simulink model "ModelRiki"  (R2020a)
settings: Solver=ode45  StartTime=0.0  StopTime=inf  MaxStep=Ts  RelTol=1e-3  EnableMultiTasking=on
model workspace (MAT data in the model file):
  CG = Simulink.Parameter
  CG.Value = [0 0 0]
  CG.DataType = 'auto'
  CG.Dimensions = [1 3]
  GPSLL = Simulink.Parameter
  GPSLL.Value = [47.255 11.345]
  GPSLL.DataType = 'auto'
  GPSLL.Dimensions = [1 2]
  Inertia = Simulink.Parameter
  Inertia.Value = [0.035  0  0; 0  0.035  0; 0  0  0.011]
  Inertia.DataType = 'auto'
  Inertia.Dimensions = [3 3]
  Mass = Simulink.Parameter
  Mass.Value = 1.6
  Mass.DataType = 'auto'
  Mass.Dimensions = [1 1]
  Ts = Simulink.Parameter
  Ts.Value = 0.0025
  Ts.DataType = 'auto'
  Ts.Dimensions = [1 1]
values from neighbouring files (symbols this model uses):
  AltKp = 0.03    [params.mat]
  AltRateBias = 0.65    [params.mat]
  AltRateKi = 0.01    [params.mat]
  AltRateKp = 0.05    [params.mat]
  AltRateMax = 6    [params.mat]
  FilterK = [0.01 0.01 0.01 0.01 0.01 0.01 0.01 0.01 0.01 0.01 0.01 0.01 ... (100 elements, 1x100)]    [params.mat]
  PosKp = 0.1    [params.mat]
  RollPitchKp = 10    [params.mat]
  RollPitchMax = 30    [params.mat]
  RollPitchRateKd = 5e-05    [params.mat]
  RollPitchRateKi = 0.002    [params.mat]
  RollPitchRateKp = 0.0007    [params.mat]
  RollPitchRateMax = 200    [params.mat]
  VelKi = 0.02    [params.mat]
  VelKp = 0.15    [params.mat]
  VelMax = 6    [params.mat]
  Waypts = [10 20 50 50 50 50 200 20 20 0 0 50 ... (27 elements, 9x3)]    [params.mat]
  YawKp = 3    [params.mat]
  YawRateKi = 0.000213867089849    [params.mat]
  YawRateKp = 0.00321759853461    [params.mat]
  YawRateMax = 180    [params.mat]
undefined symbols (not defined in the file or in its folder): AltRateKd, DiscIntNeverNeededParam, Earth, Receive, Send, sigbuilder_block, WGS84
libraries: simulink x50, sharedutil x8, simulink_extras x7, aerolibfltsims x5, aerolibanimutils x2, aerolibtransform2 x2, aerolibconvert2 x2, shared6dof x1, aerolibatmos2 x1
(part 1 of 4)
settings Model: Creator=User  LastModifiedBy=Ivan
settings SolverCC: InitialStep=Ts
settings DataIOCC: LimitDataPoints=on  SaveFormat=Array  ReturnWorkspaceOutputs=off
settings OptimizationCC: ZeroExternalMemoryAtStartup=off  ZeroInternalMemoryAtStartup=off  LifeSpan=Inf  EfficientTunableParamExpr=on
settings DebuggingCC: UnderspecifiedInitializationDetection=Classic  MergeDetectMultiDrivingBlocksExec=none  SolverPrmCheckMsg=warning  ParameterPrecisionLossMsg=none  AllowSymbolicDim=off  ModelReferenceExtraNoncontSigs=none  StateNameClashWarn=warning  SFUnexpectedBacktrackingDiag=warning  SFNoUnconditionalDefaultTransitionDiag=warning  SFExecutionAtInitializationDiag=none  ArithmeticOperatorsInVariantConditions=warning
settings HardwareCC: ProdBitPerPointer=32  ProdBitPerSizeT=32  ProdBitPerPtrDiffT=32  ProdIntDivRoundTo=Undefined  ProdWordSize=32  ProdHWDeviceType=Texas Instruments->TMS470
settings ModelReferenceCC: PropagateSignalLabelsOutOfModel=off
settings SFSimCC: SimUseLocalCustomCode=off  MATLABDynamicMemAlloc=off  CustomCodeUndefinedFunction=UseInterfaceOnly
settings RTWCC: SystemTargetFile=ert.tlc  TemplateMakefile=ert_default_tmf  GenerateReport=on  RTWUseLocalCustomCode=off  IncludeHyperlinkInReport=on  LaunchReport=on  TargetLang=C++  GenerateTraceInfo=on  GenerateTraceReport=on  GenerateTraceReportSl=on  GenerateTraceReportSf=on  GenerateTraceReportEml=on
settings CodeAppCC: StateflowObjectComments=on
settings ERTTargetCC: MultiwordLength=2048  GenerateSampleERTMain=on  MultiInstanceERTCode=on  CodeInterfacePackaging=C++ class  SupportNonFinite=off  RootIOFormat=Structure reference  ERTCustomFileTemplate=example_file_process.tlc  ConvertIfToSwitch=off  SuppressUnreachableDefaultCases=off
settings ConfigComp: CovMetricSettings=dw  CovHtmlReporting=on  CovSaveCumulativeToWorkspaceVar=on  CovSaveSingleToWorkspaceVar=on  CovExternalEMLEnable=off

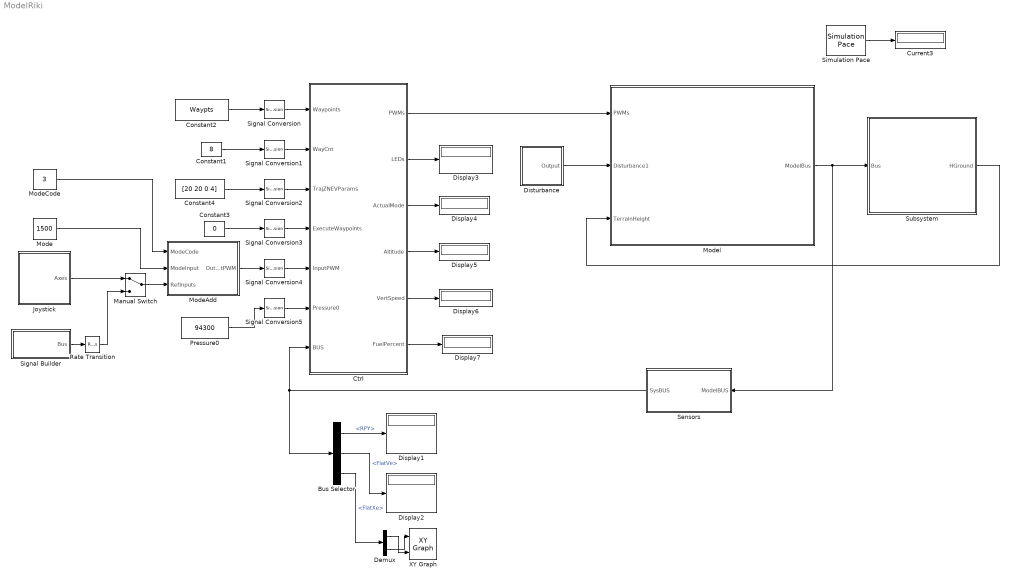
== system ModelRiki ==
  Bus Selector : BusSelector  OutputSignals=RPY,FlatVe,FlatXe
  Constant1 : Constant  Value=8  OutDataTypeStr=int32  SampleTime=Ts
  Constant2 : Constant  Value=Waypts  OutDataTypeStr=single  SampleTime=Ts
  Constant3 : Constant  Value=0  OutDataTypeStr=uint32  SampleTime=Ts
  Constant4 : Constant  Value=[20 20 0 4]  OutDataTypeStr=single  SampleTime=Ts
  Ctrl : Subsystem  TreatAsAtomicUnit=on
  Current3 : Display
  Demux : Demux  Outputs=2
  Display{1..7} (7 alike) : Display
  Disturbance : Subsystem
  Joystick : Subsystem
  Manual Switch : ManualSwitch
  Mode : Constant  Value=1500  OutDataTypeStr=uint32  SampleTime=Ts
  ModeAdd : Subsystem
  ModeCode : Constant  Value=3  OutDataTypeStr=uint8  SampleTime=Ts
  Model : Subsystem
      mask Display:
      | image('riki.jpg')
      | color('black')
      | port_label('input',1,'U')
      | port_label('input',2,'Disturbance')
      | port_label('input',3,'Terrain Height')
      | port_label('output',1,'ModelBUS')
  Pressure0 : Constant  Value=94300  OutDataTypeStr=single  SampleTime=Ts
  Rate Transition : RateTransition  OutPortSampleTime=Ts
  Sensors : Subsystem
  Signal Conversion{,1..5} (6 alike) : SignalConversion  OverrideOpt=on
  Signal Builder : Subsystem  Tag=STV Subsys  LoadFcn=sigbuilder_block('load');  StartFcn=sigbuilder_block('start');  StopFcn=sigbuilder_block('stop');  ClipboardFcn=sigbuilder_block('clipboard');  mask(Sigbuilder block){tuvar=[0:10]}
      mask help: Simulink:masks:SigbuilderBlock_MD
      mask init:
      | if ~strcmp(get_param(bdroot(gcbh),'SimulationStatus'),'stopped') tuvar = sigbuilder_block('maskInit'); end
      settings: CopyFcn=sigbuilder_block('copy');  DeleteFcn=sigbuilder_block('delete');  ModelCloseFcn=sigbuilder_block('modelClose');  PreSaveFcn=sigbuilder_block('preSave');  PauseFcn=sigbuilder_block('pause');  ContinueFcn=sigbuilder_block('continue');  NameChangeFcn=sigbuilder_block('namechange');  OpenFcn=sigbuilder_block('open',[369 90.5 830 726.5 ]);  CloseFcn=sigbuilder_block('close');
      mask Display: plot(0, 0, 100, 100,[2, 2, 32, 32, 2], [68, 8, 8, 68, 68],[32, 2], [38, 38], [32, 19, 2],[53, 60, 44], [32, 17, 17, 2],[16, 16, 31, 31]);txt = getActiveGroup(gcbh);text(2, 100, txt,'verticalAlignment', 'top');
  Simulation Pace : aerolibanimutils/Simulation Pace  SimulationPace=1  SleepMode=MATLAB Thread  OutputPaceError=on  SampleTime=Ts
      settings: AttributesFormatString=%<SimulationPace> sec/sec
  Subsystem : Subsystem
  XY Graph : simulink/Sinks/XY Graph  xmin=-100  xmax=100  ymin=-100  ymax=100  st=0.1
  wires:
  Disturbance/1(Output) -> Model/2(Disturbance1)
  Model/1(ModelBus) -> Sensors/1(ModelBUS), Subsystem/1(Bus)
  Sensors/1(SysBUS) -> Ctrl/7(BUS), Bus Selector/1
  Ctrl/1(PWMs) -> Model/1(PWMs)
  Bus Selector/1 -> Display1/1  "<RPY>"
  Ctrl/2(LEDs) -> Display3/1
  Ctrl/3(ActualMode) -> Display4/1
  Ctrl/4(Altitude) -> Display5/1
  Ctrl/5(VertSpeed) -> Display6/1
  ModeCode/1 -> ModeAdd/1(ModeCode)
  ModeAdd/1(OutputPWM) -> Signal Conversion4/1
  Subsystem/1(HGround) -> Model/3(TerrainHeight)
  Simulation Pace/1 -> Current3/1
  Bus Selector/2 -> Display2/1  "<FlatVe>"
  Mode/1 -> ModeAdd/2(ModeInput)
  Joystick/1(Axes) -> Manual Switch/1
  Manual Switch/1 -> ModeAdd/3(RefInputs)
  Constant2/1 -> Signal Conversion/1
  Constant1/1 -> Signal Conversion1/1
  Constant3/1 -> Signal Conversion3/1
  Ctrl/6(FuelPercent) -> Display7/1
  Signal Builder/1(Bus) -> Rate Transition/1
  Rate Transition/1 -> Manual Switch/2
  Demux/1 -> XY Graph/2
  Demux/2 -> XY Graph/1
  Bus Selector/3 -> Demux/1  "<FlatXe>"
  Constant4/1 -> Signal Conversion2/1
  Signal Conversion/1 -> Ctrl/1(Waypoints)
  Signal Conversion1/1 -> Ctrl/2(WayCnt)
  Signal Conversion2/1 -> Ctrl/3(TrajZNEVParams)
  Signal Conversion3/1 -> Ctrl/4(ExecuteWaypoints)
  Signal Conversion4/1 -> Ctrl/5(InputPWM)
  Pressure0/1 -> Signal Conversion5/1
  Signal Conversion5/1 -> Ctrl/6(Pressure0)

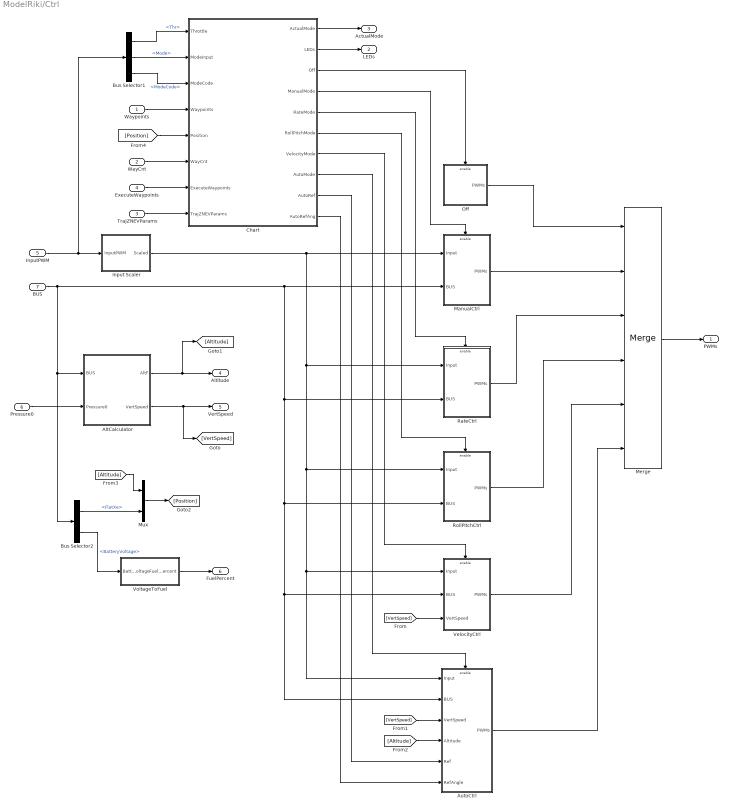
== system ModelRiki/Ctrl ==
  Waypoints : Inport
  WayCnt : Inport  Port=2
  TrajZNEVParams : Inport  Port=3
  ExecuteWaypoints : Inport  Port=4
  InputPWM : Inport  Port=5
  Pressure0 : Inport  Port=6
  BUS : Inport  Port=7
  AltCalculator : Subsystem
  AutoCtrl : Subsystem
  Bus Selector1 : BusSelector  OutputSignals=Thr,Mode,ModeCode
  Bus Selector2 : BusSelector  OutputSignals=FlatXe,BatteryVoltage
  Chart : Stateflow chart  TreatAsAtomicUnit=on
  Input Scaler : Subsystem
  ManualCtrl : Subsystem
  Merge : Merge  Inputs=6
  Mux : Mux  Inputs=2
  Off : Subsystem
  RateCtrl : Subsystem
  RollPitchCtrl : Subsystem
  VelocityCtrl : Subsystem
  VoltageToFuel : Subsystem
  PWMs : Outport
  LEDs : Outport  Port=2
  ActualMode : Outport  Port=3
  Altitude : Outport  Port=4
  VertSpeed : Outport  Port=5
  FuelPercent : Outport  Port=6
  wires:
  BUS/1 -> Bus Selector2/1, AltCalculator/1(BUS), ManualCtrl/2(BUS), RateCtrl/2(BUS), RollPitchCtrl/2(BUS), VelocityCtrl/2(BUS), AutoCtrl/2(BUS)
  InputPWM/1 -> Input Scaler/1(InputPWM), Bus Selector1/1
  Off/1(PWMs) -> Merge/1
  ManualCtrl/1(PWMs) -> Merge/2
  Merge/1 -> PWMs/1
  Chart/3(" Off") -> Off/Enable
  Chart/5(" RateMode") -> RateCtrl/Enable
  Bus Selector1/1 -> Chart/1(Throttle)  "<Thr>"
  Input Scaler/1(Scaled) -> ManualCtrl/1(Input), RateCtrl/1(Input), RollPitchCtrl/1(Input), AutoCtrl/1(Input), VelocityCtrl/1(Input)
  Chart/1(ActualMode) -> ActualMode/1
  Chart/6(" RollPitchMode") -> RollPitchCtrl/Enable
  Chart/2(LEDs) -> LEDs/1
  RollPitchCtrl/1(PWMs) -> Merge/4
  Chart/4(" ManualMode") -> ManualCtrl/Enable
  RateCtrl/1(PWMs) -> Merge/3
  AltCalculator/1(AltF) -> [Altitude], Altitude/1
  AltCalculator/2(VertSpeed) -> [VertSpeed], VertSpeed/1
  Bus Selector1/3 -> Chart/3(ModeCode)  "<ModeCode>"
  VelocityCtrl/1(PWMs) -> Merge/5
  Chart/7(" VelocityMode") -> VelocityCtrl/Enable
  AutoCtrl/1(PWMs) -> Merge/6
  Bus Selector1/2 -> Chart/2(ModeInput)  "<Mode>"
  [VertSpeed] -> VelocityCtrl/3(VertSpeed)
  [VertSpeed] -> AutoCtrl/3(VertSpeed)
  [Altitude] -> AutoCtrl/4(Altitude)
  Waypoints/1 -> Chart/4(Waypoints)
  Bus Selector2/1 -> Mux/2  "<FlatXe>"
  [Altitude] -> Mux/1
  Mux/1 -> [Position]
  [Position] -> Chart/5(Position)
  WayCnt/1 -> Chart/6(WayCnt)
  ExecuteWaypoints/1 -> Chart/7(ExecuteWaypoints)
  Bus Selector2/2 -> VoltageToFuel/1(BattVoltage)  "<BatteryVoltage>"
  VoltageToFuel/1(FuelPercent) -> FuelPercent/1
  Pressure0/1 -> AltCalculator/2(Pressure0)
  Chart/10(AutoRefAng) -> AutoCtrl/6(RefAngle)
  TrajZNEVParams/1 -> Chart/8(TrajZNEVParams)
  Chart/8(" AutoMode") -> AutoCtrl/Enable
  Chart/9(AutoRef) -> AutoCtrl/5(Ref)

== system ModelRiki/Disturbance ==
  Mode3 : Constant  Value=[0 0 0]  OutDataTypeStr=Inherit: Inherit via back propagation  SampleTime=Ts
  Mux : Mux  Inputs=2
  Step : Step  Time=10  Before=[0 0 0]  After=[0 0 0]  SampleTime=0
  Output : Outport
  wires:
  Step/1 -> Mux/1  "F[N]"
  Mux/1 -> Output/1
  Mode3/1 -> Mux/2  "Torque"

== system ModelRiki/Joystick ==
  Bus Creator : BusCreator  Inputs=4
  Joy Scaler : Subsystem
  Joystick : Subsystem
  Terminator{,1..3} (4 alike) : Terminator
  Axes : Outport
  wires:
  Joystick/1(Roll) -> Bus Creator/1  "Roll"
  Joystick/2(Pitch) -> Bus Creator/2  "Pitch"
  Joystick/3(Yaw) -> Bus Creator/3  "Yaw"
  Joystick/4(Throttle) -> Bus Creator/4  "Throttle"
  Bus Creator/1 -> Joy Scaler/1(Joystick)
  Joystick/7(B3) -> Terminator3/1
  Joystick/6(B2) -> Terminator1/1
  Joystick/5(B1) -> Terminator/1
  Joystick/8(B4) -> Terminator2/1
  Joy Scaler/1(Scaled) -> Axes/1

== system ModelRiki/ModeAdd ==
  ModeCode : Inport
  ModeInput : Inport  Port=2
  RefInputs : Inport  Port=3
  Bus Creator : BusCreator  Inputs=6
  Bus Selector2 : BusSelector  OutputSignals=Thr,Aileron,Elevator,Rudder
  Data Type Conversion{,1..3} (4 alike) : DataTypeConversion  OutDataTypeStr=single
  OutputPWM : Outport
  wires:
  Bus Selector2/1 -> Data Type Conversion/1  "<Thr>"
  Bus Selector2/2 -> Data Type Conversion1/1  "<Aileron>"
  RefInputs/1 -> Bus Selector2/1
  Bus Selector2/3 -> Data Type Conversion2/1  "<Elevator>"
  Bus Selector2/4 -> Data Type Conversion3/1  "<Rudder>"
  ModeCode/1 -> Bus Creator/1  "ModeCode"
  Bus Creator/1 -> OutputPWM/1
  ModeInput/1 -> Bus Creator/2  "Mode"
  Data Type Conversion/1 -> Bus Creator/3  "Thr"
  Data Type Conversion1/1 -> Bus Creator/4  "Aileron"
  Data Type Conversion2/1 -> Bus Creator/5  "Elevator"
  Data Type Conversion3/1 -> Bus Creator/6  "Rudder"

== system ModelRiki/Model ==
  note: DCM:
      | Pbody = DCM*Pearth
  PWMs : Inport
  Disturbance1 : Inport  Port=2
  TerrainHeight : Inport  Port=3
  6DoF (Euler Angles) : shared6dof/6DOF (Euler Angles)  units=Metric (MKS)  mtype=Fixed  rep=Euler Angles  xme_0=[0 0 -600]  Vm_0=[0 0 0]  eul_0=[0 0 0]  pm_0=[0 0 0]  mass_0=Mass  mass_e=0.5  mass_f=2.0  inertia=Inertia  inertia_e=eye(3)  inertia_f=2*eye(3)  k_quat=1.0  vre_flag=on  abi_flag=off  aMode=aMode  xme_statename=''  Vm_statename=''  eul_statename=''  quat_statename=''  pm_statename=''  mass_statename=''
      settings: SourceProductBaseCode=AE,PW,MT,VE,VP
  Bus Creator : BusCreator  Inputs=10
  Bus Selector : BusSelector  OutputSignals=PWM1,PWM2,PWM3,PWM4
  Environment : Subsystem
  GPS&Pressure : Subsystem
  Ground : Ground
  Landing Gears : Subsystem
  Manual Switch1 : ManualSwitch
  Propulsion : Subsystem
  Rate Transition : RateTransition
  Sum : Sum  Inputs=||+-+
  Sum1 : Sum  Inputs=||+-+
  Terminator1 : Terminator
  Terminator2 : Terminator
  ModelBus : Outport
  wires:
  6DoF (Euler Angles)/1 -> Bus Creator/1  "Ve"
  6DoF (Euler Angles)/2 -> GPS&Pressure/1(Xe), Bus Creator/2  "Xe"
  6DoF (Euler Angles)/3 -> Bus Creator/3  "RPY"
  6DoF (Euler Angles)/4 -> Bus Creator/4  "DCM"
  Propulsion/2(Mxyz[Nm]) -> Sum1/1
  Propulsion/1(Fxyz[N]) -> Sum/1
  6DoF (Euler Angles)/7 -> Terminator2/1
  Sum/1 -> Manual Switch1/1
  Ground/1 -> Manual Switch1/2
  PWMs/1 -> Rate Transition/1
  Bus Selector/1 -> Propulsion/1(PWM1)  "<PWM1>"
  Bus Selector/2 -> Propulsion/2(PWM2)  "<PWM2>"
  Bus Selector/3 -> Propulsion/3(PWM3)  "<PWM3>"
  Bus Selector/4 -> Propulsion/4(PWM4)  "<PWM4>"
  Manual Switch1/1 -> 6DoF (Euler Angles)/1
  6DoF (Euler Angles)/5 -> Bus Creator/5  "Vb"
  6DoF (Euler Angles)/6 -> Bus Creator/6  "dRPY"
  Rate Transition/1 -> Bus Selector/1
  6DoF (Euler Angles)/8 -> Terminator1/1  "Accel"
  GPS&Pressure/1(GpsLL) -> Bus Creator/7  "GpsLL"
  GPS&Pressure/2(GPSHeight) -> Bus Creator/8  "GpsHeight"
  GPS&Pressure/3(PressurePa) -> Bus Creator/9  "PressurePa"
  Bus Creator/1 -> Landing Gears/1(Model Bus), Environment/1(Model Bus), ModelBus/1
  Propulsion/3(TotalCurrent[A]) -> Bus Creator/10  "TotalCurrent"
  Disturbance1/1 -> Environment/2(Disturbance)
  Sum1/1 -> 6DoF (Euler Angles)/2
  Landing Gears/1(M[Nm]) -> Sum1/3
  Landing Gears/2(F[N]) -> Sum/3
  Environment/1(M[Nm]) -> Sum1/2
  Environment/2(F[N]) -> Sum/2
  TerrainHeight/1 -> Landing Gears/2(TerrainHeight)

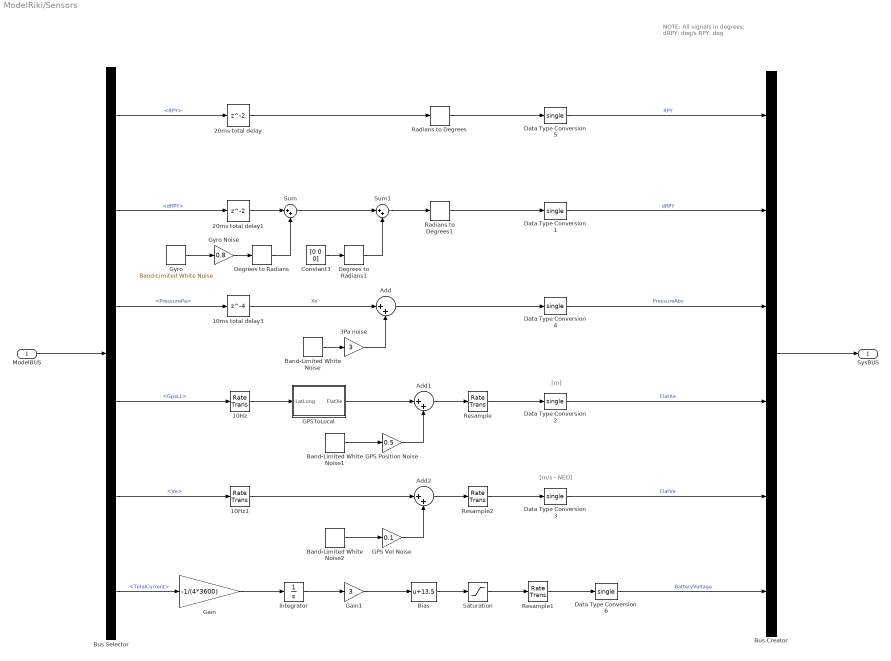
== system ModelRiki/Sensors ==
  note: [m/s - NED]
  note: [m]
  note: NOTE: All signals in degrees:
      | dRPY: deg/s
      | RPY: deg
  ModelBUS : Inport
  10Hz : RateTransition  OutPortSampleTime=1/10
  10Hz1 : RateTransition  OutPortSampleTime=1/10
  10ms total delay3 : Delay  DelayLength=4  SampleTime=Ts
  20ms total delay : Delay  SampleTime=Ts
  20ms total delay1 : Delay  SampleTime=Ts
  3Pa noise : Gain  Gain=3
  Add : Sum  Inputs=|++
  Add1 : Sum  Inputs=|++
  Add2 : Sum  Inputs=|++
  Band-Limited White Noise : simulink/Sources/Band-Limited White Noise  Cov=[1]*Ts  Ts=Ts  seed=[23341]
  Band-Limited White Noise1 : simulink/Sources/Band-Limited White Noise  Cov=[1]*Ts  Ts=Ts  seed=[23341]
  Band-Limited White Noise2 : simulink/Sources/Band-Limited White Noise  Cov=[1]*Ts  Ts=Ts  seed=[23341]
  Bias : Bias  Bias=13.5
  Bus Creator : BusCreator  Inputs=6
  Bus Selector : BusSelector  OutputSignals=RPY,dRPY,PressurePa,GpsLL,Ve,TotalCurrent
  Constant3 : Constant  Value=[0 0 0]  OutDataTypeStr=single
  Data Type Conversion{1..6} (6 alike) : DataTypeConversion  OutDataTypeStr=single
  Degrees to Radians : simulink_extras/Transformations/Degrees to Radians
  Degrees to Radians1 : simulink_extras/Transformations/Degrees to Radians
  GPS Position Noise : Gain  Gain=0.5
  GPS Vel Noise : Gain  Gain=0.1
  GPSToLocal : Subsystem
  Gain : Gain  Gain=-1/(4*3600)
  Gain1 : Gain  Gain=3
  Gyro : simulink/Sources/Band-Limited White Noise  Cov=[1]*Ts  Ts=Ts  seed=[23341]
  Gyro Noise : Gain  Gain=0.8
  Integrator : Integrator  InitialCondition=1  LimitOutput=on  UpperSaturationLimit=1  LowerSaturationLimit=0
  Radians to Degrees : simulink_extras/Transformations/Radians to Degrees
  Radians to Degrees1 : simulink_extras/Transformations/Radians to Degrees
  Resample : RateTransition  OutPortSampleTime=Ts
  Resample1 : RateTransition  OutPortSampleTime=Ts
  Resample2 : RateTransition  OutPortSampleTime=Ts
  Saturation : Saturate  UpperLimit=16.8  LowerLimit=12
  Sum : Sum  Inputs=|++
  Sum1 : Sum  Inputs=|++
  SysBUS : Outport
  wires:
  ModelBUS/1 -> Bus Selector/1
  Bus Selector/1 -> 20ms total delay/1  "<RPY>"
  Bus Creator/1 -> SysBUS/1
  Bus Selector/2 -> 20ms total delay1/1  "<dRPY>"
  20ms total delay/1 -> Radians to Degrees/1
  20ms total delay1/1 -> Sum/1
  Gyro/1 -> Gyro Noise/1
  Data Type Conversion5/1 -> Bus Creator/1  "RPY"
  Data Type Conversion1/1 -> Bus Creator/2  "dRPY"
  Degrees to Radians/1 -> Sum/2
  Radians to Degrees/1 -> Data Type Conversion5/1
  Radians to Degrees1/1 -> Data Type Conversion1/1
  Sum/1 -> Sum1/1
  Sum1/1 -> Radians to Degrees1/1
  Constant3/1 -> Degrees to Radians1/1
  Degrees to Radians1/1 -> Sum1/2
  Data Type Conversion3/1 -> Bus Creator/5  "FlatVe"
  Data Type Conversion2/1 -> Bus Creator/4  "FlatXe"
  3Pa noise/1 -> Add/2
  Band-Limited White Noise/1 -> 3Pa noise/1
  Add/1 -> Data Type Conversion4/1
  10ms total delay3/1 -> Add/1  "Xe"
  Bus Selector/3 -> 10ms total delay3/1  "<PressurePa>"
  Data Type Conversion4/1 -> Bus Creator/3  "PressureAbs"
  Bus Selector/4 -> 10Hz/1  "<GpsLL>"
  Bus Selector/5 -> 10Hz1/1  "<Ve>"
  10Hz/1 -> GPSToLocal/1(LatLong)
  Resample/1 -> Data Type Conversion2/1
  Resample2/1 -> Data Type Conversion3/1
  GPS Position Noise/1 -> Add1/2
  Band-Limited White Noise1/1 -> GPS Position Noise/1
  GPSToLocal/1(FlatXe) -> Add1/1
  Add1/1 -> Resample/1
  GPS Vel Noise/1 -> Add2/2
  Band-Limited White Noise2/1 -> GPS Vel Noise/1
  10Hz1/1 -> Add2/1
  Add2/1 -> Resample2/1
  Gyro Noise/1 -> Degrees to Radians/1
  Bus Selector/6 -> Gain/1  "<TotalCurrent>"
  Gain/1 -> Integrator/1
  Integrator/1 -> Gain1/1
  Bias/1 -> Saturation/1
  Gain1/1 -> Bias/1
  Saturation/1 -> Resample1/1
  Resample1/1 -> Data Type Conversion6/1
  Data Type Conversion6/1 -> Bus Creator/6  "BatteryVoltage"

== system ModelRiki/Signal Builder ==
  Bus Creator : BusCreator  Tag=Bus Creator  Inputs=4
  FromWs : FromWorkspace  Tag=STV FromWs  VariableName=tuvar
      SigBuilderData=|
      | common.afterFinalStr = 'Extrapolate'
      | common.sampleTime = 0
      | dataSet.timeRange = [0 20]
      | dataSet.name = 'Group 1'
      | sbobj.Groups.Name = 'Group 1'
      | sbobj.Groups.Signals(1).Name = 'Thr'
      | sbobj.Groups.Signals(1).XData = [0 20]
      | sbobj.Groups.Signals(1).YData = [1430 1430]
      | sbobj.Groups.Signals(2).Name = 'Aileron'
      | sbobj.Groups.Signals(2).XData = [0 20]
      | sbobj.Groups.Signals(2).YData = [1024 1024]
      | sbobj.Groups.Signals(3).Name = 'Elevator'
      | sbobj.Groups.Signals(3).XData = [0 20]
      | sbobj.Groups.Signals(3).YData = [1000 1000]
      | sbobj.Groups.Signals(4).Name = 'Rudder'
      | sbobj.Groups.Signals(4).XData = [0 20]
      | sbobj.Groups.Signals(4).YData = [1024 1024]
      | sbobj.Groups.TimeRange = [0 20]
  Subsystem : Subsystem
  Bus : Outport
  wires:
  FromWs/1 -> Subsystem/1(In1)
  Subsystem/1(Thr) -> Bus Creator/1  "Thr"
  Subsystem/2(Aileron) -> Bus Creator/2  "Aileron"
  Subsystem/3(Elevator) -> Bus Creator/3  "Elevator"
  Subsystem/4(Rudder) -> Bus Creator/4  "Rudder"
  Bus Creator/1 -> Bus/1

== system ModelRiki/Subsystem ==
  Bus : Inport
  Angle Conversion1 : aerolibconvert2/Angle Conversion  IU=deg  OU=rad
  Angle Conversion2 : aerolibconvert2/Angle Conversion  IU=deg  OU=rad
  Bus Selector1 : BusSelector  OutputSignals=GpsLL,GpsHeight,RPY
  Data Type Conversion1 : DataTypeConversion  OutDataTypeStr=single
  Data Type Conversion2 : DataTypeConversion  OutDataTypeStr=single
  Data Type Conversion3 : DataTypeConversion  OutDataTypeStr=single
  Demux : Demux  Outputs=2
  Demux1 : Demux  Outputs=3
  Generate Run Script : aerolibfltsims/Generate Run Script  Architecture=Win64  dataFlow=Send-Receive  GeometryModelName=Kiki  AirportId=LDZA  RunwayId=16  InitialAltitude=5000  InitialHeading=0  OffsetDistance=0  OffsetAzimuth=0  InstallScenery=off  DisableShaders=off  OriginAddress=127.0.0.1  DestinationPort=5502  OriginPort=5505  LocalAddress=127.0.0.1  OutputFileName=runfg.bat  FlightGearBaseDirectory=C:\Program Files\FlightGear 3.4.0
  Pack net_fdm Packet for FlightGear : aerolibfltsims/Pack net_fdm Packet for FlightGear  FlightGearVersion=v3.4  ShowPositionAttitudeInputs=on  ShowVelocityAccelerationInputs=off  ShowControlSurfacePositionInputs=off  ShowEngineFuelInputs=off  ShowLandingGearInputs=off  ShowEnvironmentInputs=off  SampleTime=1/30  packetVersion=24
      settings: SourceProductBaseCode=AE
  Receive net_ctrl Packet from FlightGear : aerolibfltsims/Receive net_ctrl Packet from FlightGear  FlightGearVersion=v3.4  ReceiveAddress=127.0.0.1  ReceivePort=5505  ReceiveWidth=744  varLen=off  SampleTime=1/30  packetFlag=off
      settings: AttributesFormatString=Version Selected:\n%<FlightGearVersion>  SourceProductBaseCode=AE
  Send net_fdm Packet to FlightGear : aerolibfltsims/Send net_fdm Packet to FlightGear  DestinationIpAddress=127.0.0.1  DestinationPort=5502  LocalIpPort=-1  varLen=off  SampleTime=1/30
      settings: SourceProductBaseCode=AE
  Terminator{,1..6} (7 alike) : Terminator
  Unpack net_ctrl Packet from FlightGear : aerolibfltsims/Unpack net_ctrl Packet from FlightGear  FlightGearVersion=v3.4  ShowControlSurfacePositionOutputs=off  ShowEngineFuelOutputs=off  ShowLandingGearOutputs=off  ShowAvionicOutputs=off  ShowEnvironmentOutputs=on  SampleTime=1/30  packetVersion=27
      settings: AttributesFormatString=Version Selected: %<FlightGearVersion>  SourceProductBaseCode=AE
  HGround : Outport
  wires:
  Pack net_fdm Packet for FlightGear/1 -> Send net_fdm Packet to FlightGear/1
  Bus/1 -> Bus Selector1/1
  Bus Selector1/1 -> Demux/1  "<GpsLL>"
  Demux/1 -> Angle Conversion1/1
  Demux/2 -> Angle Conversion2/1
  Bus Selector1/2 -> Pack net_fdm Packet for FlightGear/3  "<GpsHeight>"
  Demux1/1 -> Data Type Conversion1/1
  Demux1/2 -> Data Type Conversion2/1
  Demux1/3 -> Data Type Conversion3/1
  Data Type Conversion1/1 -> Pack net_fdm Packet for FlightGear/4
  Data Type Conversion2/1 -> Pack net_fdm Packet for FlightGear/5
  Data Type Conversion3/1 -> Pack net_fdm Packet for FlightGear/6
  Bus Selector1/3 -> Demux1/1  "<RPY>"
  Receive net_ctrl Packet from FlightGear/1 -> Unpack net_ctrl Packet from FlightGear/1
  Unpack net_ctrl Packet from FlightGear/6 -> HGround/1
  Angle Conversion1/1 -> Pack net_fdm Packet for FlightGear/2
  Angle Conversion2/1 -> Pack net_fdm Packet for FlightGear/1
  Unpack net_ctrl Packet from FlightGear/1 -> Terminator/1
  Unpack net_ctrl Packet from FlightGear/2 -> Terminator1/1
  Unpack net_ctrl Packet from FlightGear/3 -> Terminator2/1
  Unpack net_ctrl Packet from FlightGear/4 -> Terminator3/1
  Unpack net_ctrl Packet from FlightGear/5 -> Terminator4/1
  Unpack net_ctrl Packet from FlightGear/7 -> Terminator5/1
  Unpack net_ctrl Packet from FlightGear/8 -> Terminator6/1

== system ModelRiki/Ctrl/AltCalculator ==
  BUS : Inport
  Pressure0 : Inport  Port=2
  Bus Selector1 : BusSelector  OutputSignals=PressureAbs
  Delay : Delay  DelayLength=100
  Discrete FIR Filter : DiscreteFir  Coefficients=FilterK
  Gain : Gain  Gain=1/(100*Ts)
  MATLAB Function : MATLAB Function  TreatAsAtomicUnit=on
  Sum : Sum  Inputs=|+-
  AltF : Outport
  VertSpeed : Outport  Port=2
  wires:
  BUS/1 -> Bus Selector1/1
  Bus Selector1/1 -> MATLAB Function/1(pressure)  "<PressureAbs>"
  MATLAB Function/1(alt) -> Discrete FIR Filter/1
  Sum/1 -> Gain/1
  Discrete FIR Filter/1 -> Delay/1, Sum/1, AltF/1
  Delay/1 -> Sum/2
  Gain/1 -> VertSpeed/1
  Pressure0/1 -> MATLAB Function/2(pressure0)

== system ModelRiki/Ctrl/AutoCtrl ==
  Input : Inport  OutDataTypeStr=single
  BUS : Inport  Port=2  OutDataTypeStr=single
  VertSpeed : Inport  Port=3  OutDataTypeStr=single
  Altitude : Inport  Port=4  OutDataTypeStr=single
  Ref : Inport  Port=5  OutDataTypeStr=single
  RefAngle : Inport  Port=6  OutDataTypeStr=single
  Enable : EnablePort  StatesWhenEnabling=reset
  Alt Controller : Subsystem
  Bus Selector1 : BusSelector  OutputSignals=Rudder
  Demux : Demux  Outputs=3
  Mapper : Subsystem
  Pitch Controller : Subsystem
  Position Ctrl : Subsystem
  Roll Controller : Subsystem
  Velocity Ctrl : Subsystem
  Yaw Controller : Subsystem
  PWMs : Outport
  wires:
  BUS/1 -> Yaw Controller/1(BUS), Pitch Controller/1(BUS), Position Ctrl/1(BUS), Roll Controller/1(BUS), Velocity Ctrl/1(BUS)
  Input/1 -> Bus Selector1/1
  Bus Selector1/1 -> Yaw Controller/2(YawRef)  "<Rudder>"
  Mapper/1(Out1) -> PWMs/1
  Roll Controller/1(RollPWM) -> Mapper/2(Aileron)
  Pitch Controller/1(PitchPWM) -> Mapper/3(Elevator)
  Yaw Controller/1(YawPWM) -> Mapper/4(Rudder)
  Velocity Ctrl/1(RollRef) -> Roll Controller/2(RollRef)  "RollRef"
  Velocity Ctrl/2(PitchRef) -> Pitch Controller/2(PitchRef)  "PitchRef"
  VertSpeed/1 -> Alt Controller/2(VertVel)
  Alt Controller/1(Thrust) -> Mapper/1(Thr)
  Altitude/1 -> Alt Controller/3(Altitude)
  Position Ctrl/1(VeXref) -> Velocity Ctrl/2(VeXref)
  Position Ctrl/2(VeYRef) -> Velocity Ctrl/3(VeYref)
  Demux/2 -> Position Ctrl/2(XeXRef)
  Demux/3 -> Position Ctrl/3(XeYRef)
  Ref/1 -> Demux/1
  Demux/1 -> Alt Controller/1(AltRef)
  RefAngle/1 -> Yaw Controller/3(RefAngle)

== system ModelRiki/Ctrl/Input Scaler ==
  InputPWM : Inport
  Bus Creator : BusCreator  Inputs=4
  Bus Selector2 : BusSelector  OutputSignals=Thr,Aileron,Elevator,Rudder
  Constant : Constant  Value=350  OutDataTypeStr=single
  Constant1 : Constant  Value=1024  OutDataTypeStr=single
  Constant2 : Constant  Value=1024  OutDataTypeStr=single
  Constant3 : Constant  Value=1024  OutDataTypeStr=single
  Gain : Gain  Gain=1/(1700-350)
  Gain1 : Gain  Gain=-1/(1700-1024)
  Gain2 : Gain  Gain=-1/(1700-1024)
  Gain3 : Gain  Gain=-1/(1700-1024)
  Saturation : Saturate  UpperLimit=1  LowerLimit=0
  Saturation1 : Saturate  UpperLimit=1  LowerLimit=-1
  Saturation2 : Saturate  UpperLimit=1  LowerLimit=-1
  Saturation3 : Saturate  UpperLimit=1  LowerLimit=-1
  Subtract{,1..3} (4 alike) : Sum  Inputs=+-
  Scaled : Outport
  wires:
  Bus Creator/1 -> Scaled/1
  InputPWM/1 -> Bus Selector2/1
  Bus Selector2/1 -> Subtract/1  "<Thr>"
  Constant/1 -> Subtract/2
  Subtract/1 -> Gain/1
  Gain/1 -> Saturation/1
  Saturation/1 -> Bus Creator/1  "Thr"
  Bus Selector2/2 -> Subtract1/1  "<Aileron>"
  Constant1/1 -> Subtract1/2
  Subtract1/1 -> Gain1/1
  Gain1/1 -> Saturation1/1
  Saturation1/1 -> Bus Creator/2  "Aileron"
  Bus Selector2/3 -> Subtract2/1  "<Elevator>"
  Constant2/1 -> Subtract2/2
  Subtract2/1 -> Gain2/1
  Gain2/1 -> Saturation2/1
  Saturation2/1 -> Bus Creator/3  "Elevator"
  Bus Selector2/4 -> Subtract3/1  "<Rudder>"
  Constant3/1 -> Subtract3/2
  Subtract3/1 -> Gain3/1
  Gain3/1 -> Saturation3/1
  Saturation3/1 -> Bus Creator/4  "Rudder"

== system ModelRiki/Ctrl/ManualCtrl ==
  Input : Inport  OutDataTypeStr=single
  BUS : Inport  Port=2  OutDataTypeStr=single
  Enable : EnablePort  StatesWhenEnabling=reset
  Bus Selector1 : BusSelector  OutputSignals=Thr,Aileron,Elevator,Rudder
  Gain : Gain
  Gain1 : Gain  Gain=0.2
  Gain2 : Gain  Gain=0.2
  Gain3 : Gain  Gain=0.2
  Mapper : Subsystem
  Terminator : Terminator
  PWMs : Outport
  wires:
  Bus Selector1/4 -> Gain3/1  "<Rudder>"
  Input/1 -> Bus Selector1/1
  Bus Selector1/1 -> Gain/1  "<Thr>"
  Bus Selector1/3 -> Gain2/1  "<Elevator>"
  Bus Selector1/2 -> Gain1/1  "<Aileron>"
  BUS/1 -> Terminator/1
  Gain/1 -> Mapper/1(Thr)
  Gain1/1 -> Mapper/2(Aileron)
  Gain2/1 -> Mapper/3(Elevator)
  Gain3/1 -> Mapper/4(Rudder)
  Mapper/1(Out1) -> PWMs/1

== system ModelRiki/Ctrl/Off ==
  Enable : EnablePort  StatesWhenEnabling=reset
  Bus Creator : BusCreator  Inputs=4
  Constant{1..4} (4 alike) : Constant  Value=1000  OutDataTypeStr=single  SampleTime=Ts
  PWMs : Outport  InitialOutput=[1000 1000 1000 1000]
  wires:
  Bus Creator/1 -> PWMs/1
  Constant2/1 -> Bus Creator/1  "PWM1"
  Constant1/1 -> Bus Creator/2  "PWM2"
  Constant4/1 -> Bus Creator/4  "PWM4"
  Constant3/1 -> Bus Creator/3  "PWM3"

== system ModelRiki/Ctrl/RateCtrl ==
  Input : Inport  OutDataTypeStr=single
  BUS : Inport  Port=2  OutDataTypeStr=single
  Enable : EnablePort  StatesWhenEnabling=reset
  Bus Selector1 : BusSelector  OutputSignals=Thr,Aileron,Elevator,Rudder
  Gain : Gain
  Mapper : Subsystem
  Pitch Controller : Subsystem
  Roll Controller : Subsystem
  Yaw Controller : Subsystem
  PWMs : Outport
  wires:
  Bus Selector1/4 -> Yaw Controller/2(YawRef)  "<Rudder>"
  Input/1 -> Bus Selector1/1
  Bus Selector1/1 -> Gain/1  "<Thr>"
  Bus Selector1/3 -> Pitch Controller/2(PitchRef)  "<Elevator>"
  Bus Selector1/2 -> Roll Controller/2(RollRef)  "<Aileron>"
  BUS/1 -> Roll Controller/1(BUS), Pitch Controller/1(BUS), Yaw Controller/1(BUS)
  Mapper/1(Out1) -> PWMs/1
  Gain/1 -> Mapper/1(Thr)
  Roll Controller/1(RollPWM) -> Mapper/2(Aileron)
  Pitch Controller/1(PitchPWM) -> Mapper/3(Elevator)
  Yaw Controller/1(YawPWM) -> Mapper/4(Rudder)

== system ModelRiki/Ctrl/RollPitchCtrl ==
  Input : Inport  OutDataTypeStr=single
  BUS : Inport  Port=2  OutDataTypeStr=single
  Enable : EnablePort  StatesWhenEnabling=reset
  Bus Selector1 : BusSelector  OutputSignals=Thr,Aileron,Elevator,Rudder
  Gain : Gain
  Mapper : Subsystem
  Pitch Controller : Subsystem
  Roll Controller : Subsystem
  Yaw Controller : Subsystem
  PWMs : Outport
  wires:
  Bus Selector1/4 -> Yaw Controller/2(YawRef)  "<Rudder>"
  Input/1 -> Bus Selector1/1
  Bus Selector1/1 -> Gain/1  "<Thr>"
  Bus Selector1/3 -> Pitch Controller/2(PitchRef)  "<Elevator>"
  Bus Selector1/2 -> Roll Controller/2(RollRef)  "<Aileron>"
  BUS/1 -> Roll Controller/1(BUS), Yaw Controller/1(BUS), Pitch Controller/1(BUS)
  Mapper/1(Out1) -> PWMs/1
  Gain/1 -> Mapper/1(Thr)
  Roll Controller/1(RollPWM) -> Mapper/2(Aileron)
  Pitch Controller/1(PitchPWM) -> Mapper/3(Elevator)
  Yaw Controller/1(YawPWM) -> Mapper/4(Rudder)

== system ModelRiki/Ctrl/VelocityCtrl ==
  Input : Inport  OutDataTypeStr=single
  BUS : Inport  Port=2  OutDataTypeStr=single
  VertSpeed : Inport  Port=3  OutDataTypeStr=single
  Enable : EnablePort  StatesWhenEnabling=reset
  Alt Controller : Subsystem
  Bus Selector1 : BusSelector  OutputSignals=Thr,Elevator,Aileron,Rudder
  Gain2 : Gain  Gain=-1
  Mapper : Subsystem
  Pitch Controller : Subsystem
  Roll Controller : Subsystem
  Velocity Ctrl1 : Subsystem
  Yaw Controller : Subsystem
  PWMs : Outport
  wires:
  BUS/1 -> Velocity Ctrl1/1(BUS), Yaw Controller/1(BUS), Pitch Controller/1(BUS), Roll Controller/1(BUS)
  Input/1 -> Bus Selector1/1
  Bus Selector1/4 -> Yaw Controller/2(YawRef)  "<Rudder>"
  Roll Controller/1(RollPWM) -> Mapper/2(Aileron)
  Pitch Controller/1(PitchPWM) -> Mapper/3(Elevator)
  Yaw Controller/1(YawPWM) -> Mapper/4(Rudder)
  Bus Selector1/3 -> Velocity Ctrl1/3(VeYref)  "<Aileron>"
  Bus Selector1/2 -> Gain2/1  "<Elevator>"
  Velocity Ctrl1/1(RollRef) -> Roll Controller/2(RollRef)  "RollRef"
  Velocity Ctrl1/2(PitchRef) -> Pitch Controller/2(PitchRef)  "PitchRef"
  Gain2/1 -> Velocity Ctrl1/2(VeXref)
  Bus Selector1/1 -> Alt Controller/1(VertVellRef)  "<Thr>"
  VertSpeed/1 -> Alt Controller/2(VertVel)
  Alt Controller/1(Thrust) -> Mapper/1(Thr)
  Mapper/1(Out1) -> PWMs/1

== system ModelRiki/Ctrl/VoltageToFuel ==
  BattVoltage : Inport
  Polynomial : Polyval  Coefs=[-20.235749769635976 666.2775704118918 -5384.291364540743]
  Saturation : Saturate  UpperLimit=16.5  LowerLimit=14
  Saturation1 : Saturate  UpperLimit=100  LowerLimit=0
  FuelPercent : Outport
  wires:
  BattVoltage/1 -> Saturation/1
  Polynomial/1 -> Saturation1/1
  Saturation1/1 -> FuelPercent/1
  Saturation/1 -> Polynomial/1

== system ModelRiki/Joystick/Joy Scaler ==
  Joystick : Inport
  Bus Creator : BusCreator  Inputs=4
  Bus Selector2 : BusSelector  OutputSignals=Throttle,Roll,Pitch,Yaw
  Constant : Constant  Value=350  OutDataTypeStr=single
  Constant1 : Constant  Value=1024  OutDataTypeStr=single
  Constant2 : Constant  Value=1024  OutDataTypeStr=single
  Constant3 : Constant  Value=1024  OutDataTypeStr=single
  Gain : Gain  Gain=(1700-350)
  Gain1 : Gain  Gain=-(1024-350)
  Gain2 : Gain  Gain=-(1024-350)
  Gain3 : Gain  Gain=-(1024-350)
  Saturation{,1..3} (4 alike) : Saturate  UpperLimit=1700  LowerLimit=350  OutDataTypeStr=Inherit: Inherit via back propagation
  Subtract{,1..3} (4 alike) : Sum
  Scaled : Outport
  wires:
  Bus Creator/1 -> Scaled/1
  Joystick/1 -> Bus Selector2/1
  Bus Selector2/1 -> Gain/1  "<Throttle>"
  Constant/1 -> Subtract/2
  Saturation/1 -> Bus Creator/1  "Thr"
  Gain/1 -> Subtract/1
  Subtract/1 -> Saturation/1
  Constant1/1 -> Subtract1/2
  Saturation1/1 -> Bus Creator/2  "Aileron"
  Gain1/1 -> Subtract1/1
  Subtract1/1 -> Saturation1/1
  Bus Selector2/2 -> Gain1/1  "<Roll>"
  Constant2/1 -> Subtract2/2
  Saturation2/1 -> Bus Creator/3  "Elevator"
  Gain2/1 -> Subtract2/1
  Subtract2/1 -> Saturation2/1
  Bus Selector2/3 -> Gain2/1  "<Pitch>"
  Constant3/1 -> Subtract3/2
  Saturation3/1 -> Bus Creator/4  "Rudder"
  Gain3/1 -> Subtract3/1
  Subtract3/1 -> Saturation3/1
  Bus Selector2/4 -> Gain3/1  "<Yaw>"

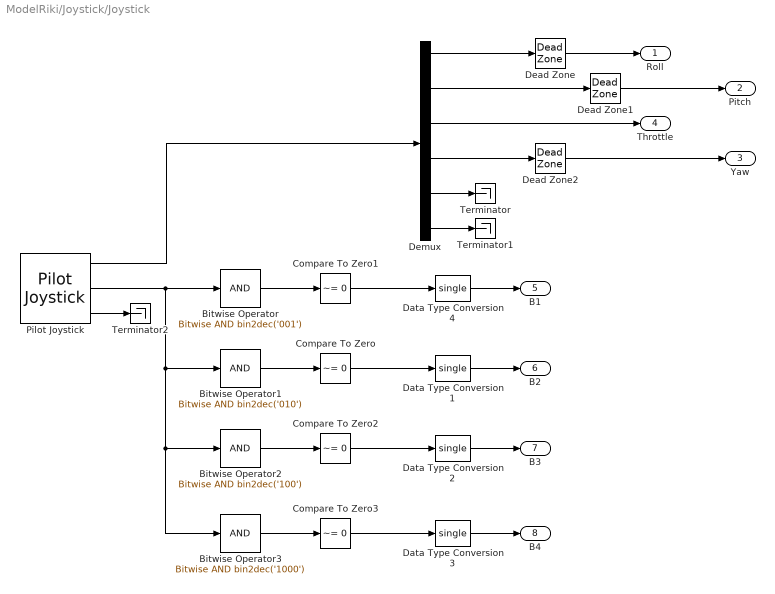
== system ModelRiki/Joystick/Joystick ==
  Bitwise Operator : simulink/Logic and Bit Operations/Bitwise Operator  logicop=AND  UseBitMask=on  BitMask=bin2dec('001')  BitMaskRealWorld=Stored Integer
  Bitwise Operator1 : simulink/Logic and Bit Operations/Bitwise Operator  logicop=AND  UseBitMask=on  BitMask=bin2dec('010')  BitMaskRealWorld=Stored Integer
  Bitwise Operator2 : simulink/Logic and Bit Operations/Bitwise Operator  logicop=AND  UseBitMask=on  BitMask=bin2dec('100')  BitMaskRealWorld=Stored Integer
  Bitwise Operator3 : simulink/Logic and Bit Operations/Bitwise Operator  logicop=AND  UseBitMask=on  BitMask=bin2dec('1000')  BitMaskRealWorld=Stored Integer
  Compare To Zero{,1..3} (4 alike) : simulink/Logic and Bit Operations/Compare To Zero  relop=~=  OutDataTypeStr=uint8
  Data Type Conversion{1..4} (4 alike) : DataTypeConversion  OutDataTypeStr=single
  Dead Zone : DeadZone  LowerValue=-0.12  UpperValue=0.12  SaturateOnIntegerOverflow=on
  Dead Zone1 : DeadZone  LowerValue=-0.12  UpperValue=0.12  SaturateOnIntegerOverflow=on
  Dead Zone2 : DeadZone  LowerValue=-0.12  UpperValue=0.12  SaturateOnIntegerOverflow=on
  Demux : Demux  Outputs=6
  Pilot Joystick : aerolibanimutils/Pilot Joystick  JoystickID=Joystick1  OutputConfiguration=AllOutputs  SampleTime=Ts
  Terminator : Terminator
  Terminator1 : Terminator
  Terminator2 : Terminator
  Roll : Outport
  Pitch : Outport  Port=2
  Yaw : Outport  Port=3
  Throttle : Outport  Port=4
  B1 : Outport  Port=5
  B2 : Outport  Port=6
  B3 : Outport  Port=7
  B4 : Outport  Port=8
  wires:
  Pilot Joystick/2 -> Bitwise Operator/1, Bitwise Operator1/1, Bitwise Operator2/1, Bitwise Operator3/1
  Demux/1 -> Dead Zone/1
  Demux/2 -> Dead Zone1/1
  Demux/4 -> Dead Zone2/1
  Demux/3 -> Throttle/1
  Bitwise Operator/1 -> Compare To Zero1/1
  Bitwise Operator1/1 -> Compare To Zero/1
  Compare To Zero/1 -> Data Type Conversion1/1
  Bitwise Operator2/1 -> Compare To Zero2/1
  Compare To Zero2/1 -> Data Type Conversion2/1
  Bitwise Operator3/1 -> Compare To Zero3/1
  Compare To Zero3/1 -> Data Type Conversion3/1
  Data Type Conversion1/1 -> B2/1
  Data Type Conversion2/1 -> B3/1
  Data Type Conversion3/1 -> B4/1
  Compare To Zero1/1 -> Data Type Conversion4/1
  Data Type Conversion4/1 -> B1/1
  Pilot Joystick/1 -> Demux/1
  Demux/6 -> Terminator1/1
  Demux/5 -> Terminator/1
  Pilot Joystick/3 -> Terminator2/1
  Dead Zone/1 -> Roll/1
  Dead Zone1/1 -> Pitch/1
  Dead Zone2/1 -> Yaw/1

== system ModelRiki/Model/Environment ==
  Model Bus : Inport
  Disturbance : Inport  Port=2
  Bus Selector : BusSelector  OutputSignals=DCM,Vb,dRPY
  Demux : Demux  Outputs=2
  Gravity : Subsystem
  Gyro dampener : Gain  Gain=0
  Sum : Sum
  Sum1 : Sum  Inputs=|++
  Sum2 : Sum  Inputs=|++
  Vel. dampener : Gain  Gain=[0 0 0]
  M[Nm] : Outport
  F[N] : Outport  Port=2
  wires:
  Model Bus/1 -> Bus Selector/1
  Bus Selector/1 -> Gravity/1(DCM)  "<DCM>"
  Bus Selector/3 -> Gyro dampener/1  "<dRPY>"
  Bus Selector/2 -> Vel. dampener/1  "<Vb>"
  Gravity/1(F[N]) -> Sum/1
  Vel. dampener/1 -> Sum/2
  Sum/1 -> Sum2/1
  Sum2/1 -> F[N]/1
  Gyro dampener/1 -> Sum1/1
  Sum1/1 -> M[Nm]/1
  Disturbance/1 -> Demux/1
  Demux/1 -> Sum2/2
  Demux/2 -> Sum1/2

== system ModelRiki/Model/GPS&Pressure ==
  Xe : Inport
  COESA Atmosphere Model : aerolibatmos2/COESA Atmosphere Model  units=Metric (MKS)  spec=1976 COESA-extended U.S. Standard Atmosphere  model=Profile  profile_var=High temperature  profile_percent=1%  profile_alt=5 km (16404 ft)  envelope_var=High temperature  envelope_percent=1%  action=Warning
  Constant : Constant  Value=0
  Flat Earth to LLA : aerolibtransform2/Flat Earth to LLA  units=Metric (MKS)  ptype=Earth (WGS84)  F=1/298.257223563  R=6378137  refPosPort=off  LL0=GPSLL  psi=0
  Invert : Gain  Gain=-1
  Selector1 : Selector  InputPortWidth=3  IndexOptions=Index vector (dialog)  Indices=[3]  OutputSizes=1
  Terminator : Terminator
  Terminator3 : Terminator
  Terminator4 : Terminator
  GpsLL : Outport
  GPSHeight : Outport  Port=2
  PressurePa : Outport  Port=3
  wires:
  COESA Atmosphere Model/4 -> Terminator4/1
  COESA Atmosphere Model/2 -> Terminator3/1
  Xe/1 -> Flat Earth to LLA/1, Selector1/1
  Invert/1 -> COESA Atmosphere Model/1
  Selector1/1 -> Invert/1
  COESA Atmosphere Model/1 -> Terminator/1
  Flat Earth to LLA/1 -> GpsLL/1  "GpsLL"
  COESA Atmosphere Model/3 -> PressurePa/1  "PressurePa"
  Flat Earth to LLA/2 -> GPSHeight/1  "GPSHeight"
  Constant/1 -> Flat Earth to LLA/2

== system ModelRiki/Model/Landing Gears ==
  Model Bus : Inport
  TerrainHeight : Inport  Port=2
  Sum1 : Sum  Inputs=++++
  Sum3 : Sum  Inputs=++++
  W1 Wheel : Subsystem  mask{WheelLoc=[0.15 -0.15 0.1]}
      mask prompts: WheelLoc "Wheel Location"
  W2 Wheel : Subsystem  mask{WheelLoc=[0.15 0.15 0.1]}
      mask prompts: WheelLoc "Wheel Location"
  W3 Wheel : Subsystem  mask{WheelLoc=[-0.15 0.15 0.1]}
      mask prompts: WheelLoc "Wheel Location"
  W4 Wheel : Subsystem  mask{WheelLoc=[-0.15 -0.15 0.1]}
      mask prompts: WheelLoc "Wheel Location"
  M[Nm] : Outport
  F[N] : Outport  Port=2
  wires:
  Model Bus/1 -> W4 Wheel/1(Model BUS), W3 Wheel/1(Model BUS), W1 Wheel/1(Model BUS), W2 Wheel/1(Model BUS)
  Sum3/1 -> M[Nm]/1
  Sum1/1 -> F[N]/1
  W1 Wheel/1(M[Nm]) -> Sum3/1
  W1 Wheel/2(F[N]) -> Sum1/1
  W3 Wheel/1(M[Nm]) -> Sum3/3
  W2 Wheel/1(M[Nm]) -> Sum3/2
  W2 Wheel/2(F[N]) -> Sum1/2
  W3 Wheel/2(F[N]) -> Sum1/3
  W4 Wheel/1(M[Nm]) -> Sum3/4
  W4 Wheel/2(F[N]) -> Sum1/4
  TerrainHeight/1 -> W1 Wheel/2(TerrainHeight), W2 Wheel/2(TerrainHeight), W3 Wheel/2(TerrainHeight), W4 Wheel/2(TerrainHeight)

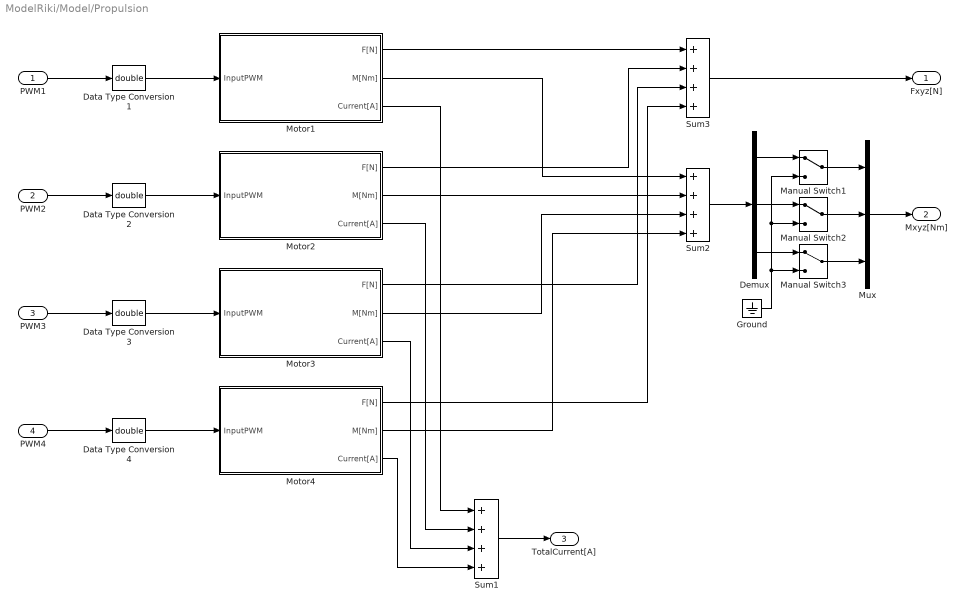
== system ModelRiki/Model/Propulsion ==
  PWM1 : Inport
  PWM2 : Inport  Port=2
  PWM3 : Inport  Port=3
  PWM4 : Inport  Port=4
  Data Type Conversion{1..4} (4 alike) : DataTypeConversion  OutDataTypeStr=double
  Demux : Demux  Outputs=3
  Ground : Ground
  Manual Switch1 : ManualSwitch
  Manual Switch2 : ManualSwitch
  Manual Switch3 : ManualSwitch
  Motor1 : Subsystem
  Motor2 : Subsystem
  Motor3 : Subsystem
  Motor4 : Subsystem
  Mux : Mux  Inputs=3
  Sum1 : Sum  Inputs=++++
  Sum2 : Sum  Inputs=++++
  Sum3 : Sum  Inputs=++++
  Fxyz[N] : Outport
  Mxyz[Nm] : Outport  Port=2
  TotalCurrent[A] : Outport  Port=3
  wires:
  Sum3/1 -> Fxyz[N]/1
  Manual Switch1/1 -> Mux/1
  Manual Switch2/1 -> Mux/2
  Manual Switch3/1 -> Mux/3
  Demux/1 -> Manual Switch1/1
  Demux/3 -> Manual Switch3/1
  Demux/2 -> Manual Switch2/1
  Sum2/1 -> Demux/1
  Mux/1 -> Mxyz[Nm]/1
  Ground/1 -> Manual Switch1/2, Manual Switch2/2, Manual Switch3/2
  Motor1/1(F[N]) -> Sum3/1
  Motor1/2(M[Nm]) -> Sum2/1
  PWM1/1 -> Data Type Conversion1/1
  PWM2/1 -> Data Type Conversion2/1
  PWM3/1 -> Data Type Conversion3/1
  PWM4/1 -> Data Type Conversion4/1
  Motor2/1(F[N]) -> Sum3/2
  Motor3/1(F[N]) -> Sum3/3
  Motor4/1(F[N]) -> Sum3/4
  Motor2/2(M[Nm]) -> Sum2/2
  Motor3/2(M[Nm]) -> Sum2/3
  Motor4/2(M[Nm]) -> Sum2/4
  Data Type Conversion1/1 -> Motor1/1(InputPWM)
  Data Type Conversion2/1 -> Motor2/1(InputPWM)
  Data Type Conversion3/1 -> Motor3/1(InputPWM)
  Data Type Conversion4/1 -> Motor4/1(InputPWM)
  Motor1/3(Current[A]) -> Sum1/1
  Motor4/3(Current[A]) -> Sum1/4
  Motor2/3(Current[A]) -> Sum1/2
  Motor3/3(Current[A]) -> Sum1/3
  Sum1/1 -> TotalCurrent[A]/1

== system ModelRiki/Sensors/GPSToLocal ==
  LatLong : Inport
  Constant : Constant  Value=0
  LLA to Flat Earth : aerolibtransform2/LLA to Flat Earth  units=Metric (MKS)  ptype=Earth (WGS84)  F=1/298.257223563  R=6378137  refPosPort=off  LL0=GPSLL  psi=0
      settings: SourceProductBaseCode=AE
  Selector : Selector  InputPortWidth=3  IndexOptions=Index vector (dialog)  Indices=[1 2]  OutputSizes=1
  FlatXe : Outport
  wires:
  LatLong/1 -> LLA to Flat Earth/1
  Constant/1 -> LLA to Flat Earth/2, LLA to Flat Earth/3
  LLA to Flat Earth/1 -> Selector/1
  Selector/1 -> FlatXe/1

== system ModelRiki/Signal Builder/Subsystem ==
  In1 : Inport
  Demux : Demux  Tag=STV Demux
      settings: DisplayOption=none
  Thr : Outport  Tag=STV Outport
  Aileron : Outport  Tag=STV Outport  Port=2
  Elevator : Outport  Tag=STV Outport  Port=3
  Rudder : Outport  Tag=STV Outport  Port=4
  wires:
  Demux/1 -> Thr/1
  Demux/2 -> Aileron/1
  Demux/3 -> Elevator/1
  Demux/4 -> Rudder/1
  In1/1 -> Demux/1

== system ModelRiki/Ctrl/AutoCtrl/Alt Controller ==
  AltRef : Inport
  VertVel : Inport  Port=2
  Altitude : Inport  Port=3
  Bias1 : Bias  Bias=AltRateBias
  Discrete PID Controller1 : simulink/Continuous/PID Controller  Controller=PI  Form=Parallel  TimeDomain=Discrete-time  UseExternalTs=off  SampleTime=Ts  IntegratorMethod=Forward Euler  FilterMethod=Forward Euler  ControllerParametersSource=internal  P=AltRateKp  I=AltRateKi  D=0  UseFilter=on  N=50  TunerSelectOption=Transfer Function Based (PID Tuner App)  InitialConditionSource=internal  InitialConditionForIntegrator=0  InitialConditionForFilter=0  DifferentiatorICPrevScaledInput=0  ExternalReset=none  TrackingMode=off  Kt=1  LimitOutput=on  UpperSaturationLimit=0.4  LowerSaturationLimit=-0.4  LinearizeAsGain=off  AntiWindupMode=clamping  Kb=1  POutMin=[]  POutMax=[]  IOutMin=[]  IOutMax=[]  DOutMin=[]  DOutMax=[]  NOutMin=[]  NOutMax=[]  SumOutMin=[]  SumOutMax=[]  SaturationOutMin=[]  SaturationOutMax=[]  PParamMin=[]  PParamMax=[]  IParamMin=[]  IParamMax=[]  DParamMin=[]  DParamMax=[]  NParamMin=[]  NParamMax=[]  KbParamMin=[]  KbParamMax=[]  KtParamMin=[]  KtParamMax=[]  KbOutMin=[]  KbOutMax=[]  KtOutMin=[]  KtOutMax=[]  IntegratorOutMin=[]  IntegratorOutMax=[]  FilterOutMin=[]  FilterOutMax=[]  SumI1OutMin=[]  SumI1OutMax=[]  SumI2OutMin=[]  SumI2OutMax=[]  SumI3OutMin=[]  SumI3OutMax=[]  SumI4OutMin=[]  SumI4OutMax=[]  SumDOutMin=[]  SumDOutMax=[]  DifferentiatorOutMin=[]  DifferentiatorOutMax=[]  FilterDiffOutCoefMin=[]  FilterDiffOutCoefMax=[]  ReciprocalOutMin=[]  ReciprocalOutMax=[]  SumDenOutMin=[]  SumDenOutMax=[]  SumNumOutMin=[]  SumNumOutMax=[]  DivideOutMin=[]  DivideOutMax=[]  UdiffTsProdOutMin=[]  UdiffTsProdOutMax=[]  NTsProdOutMin=[]  NTsProdOutMax=[]  UintegralTsProdOutMin=[]  UintegralTsProdOutMax=[]  UngainTsProdOutMin=[]  UngainTsProdOutMax=[]  IntegratorContinuousStateAttributes=''  IntegratorStateMustResolveToSignalObject=off  IntegratorRTWStateStorageClass=Auto  FilterContinuousStateAttributes=''  FilterStateMustResolveToSignalObject=off  FilterRTWStateStorageClass=Auto  ParallelPVariant=InternalParameters  IdealPVariant=Disabled  IVariant=InternalParameters  DVariant=Disabled  IntegratorVariant=Discrete  SatVariant=Enabled  AWVariant=DiscClampingParallel  PCopyVariant=Disabled  TRVariant=Disabled  FdbkBlocksVariant=Forward  IdealPFdbkVariant=Disabled  SatFdbkVariant=Disabled  DerivativeFilterVariant=Disabled  NVariant=Disabled  NCopyVariant=Disabled_SignalSpec  FilterICVariant=Disabled  IntegratorICVariant=InternalICs  ExternalResetVariant=Disabled  TRSumVariant=Passthrough  SumFdbkVariant=Disabled  SumVariant=Sum_PI  TsampFilterVariant=InternalTs  TsampNgainVariant=Passthrough  TsampIntegralVariant=Passthrough
  Discrete PID Controller2 : simulink/Continuous/PID Controller  Controller=P  Form=Parallel  TimeDomain=Discrete-time  UseExternalTs=off  SampleTime=Ts  IntegratorMethod=Forward Euler  FilterMethod=Forward Euler  ControllerParametersSource=internal  P=AltKp  I=AltRateKi  D=0  UseFilter=on  N=50  TunerSelectOption=Transfer Function Based (PID Tuner App)  InitialConditionSource=internal  InitialConditionForIntegrator=0  InitialConditionForFilter=0  DifferentiatorICPrevScaledInput=0  ExternalReset=none  TrackingMode=off  Kt=1  LimitOutput=on  UpperSaturationLimit=0.5  LowerSaturationLimit=-0.5  LinearizeAsGain=off  AntiWindupMode=clamping  Kb=1  POutMin=[]  POutMax=[]  IOutMin=[]  IOutMax=[]  DOutMin=[]  DOutMax=[]  NOutMin=[]  NOutMax=[]  SumOutMin=[]  SumOutMax=[]  SaturationOutMin=[]  SaturationOutMax=[]  PParamMin=[]  PParamMax=[]  IParamMin=[]  IParamMax=[]  DParamMin=[]  DParamMax=[]  NParamMin=[]  NParamMax=[]  KbParamMin=[]  KbParamMax=[]  KtParamMin=[]  KtParamMax=[]  KbOutMin=[]  KbOutMax=[]  KtOutMin=[]  KtOutMax=[]  IntegratorOutMin=[]  IntegratorOutMax=[]  FilterOutMin=[]  FilterOutMax=[]  SumI1OutMin=[]  SumI1OutMax=[]  SumI2OutMin=[]  SumI2OutMax=[]  SumI3OutMin=[]  SumI3OutMax=[]  SumI4OutMin=[]  SumI4OutMax=[]  SumDOutMin=[]  SumDOutMax=[]  DifferentiatorOutMin=[]  DifferentiatorOutMax=[]  FilterDiffOutCoefMin=[]  FilterDiffOutCoefMax=[]  ReciprocalOutMin=[]  ReciprocalOutMax=[]  SumDenOutMin=[]  SumDenOutMax=[]  SumNumOutMin=[]  SumNumOutMax=[]  DivideOutMin=[]  DivideOutMax=[]  UdiffTsProdOutMin=[]  UdiffTsProdOutMax=[]  NTsProdOutMin=[]  NTsProdOutMax=[]  UintegralTsProdOutMin=[]  UintegralTsProdOutMax=[]  UngainTsProdOutMin=[]  UngainTsProdOutMax=[]  IntegratorContinuousStateAttributes=''  IntegratorStateMustResolveToSignalObject=off  IntegratorRTWStateStorageClass=Auto  FilterContinuousStateAttributes=''  FilterStateMustResolveToSignalObject=off  FilterRTWStateStorageClass=Auto  ParallelPVariant=InternalParameters  IdealPVariant=Disabled  IVariant=Disabled  DVariant=Disabled  IntegratorVariant=Disabled  SatVariant=Enabled  AWVariant=Disabled  PCopyVariant=Disabled  TRVariant=Disabled  FdbkBlocksVariant=Forward  IdealPFdbkVariant=Disabled  SatFdbkVariant=Disabled  DerivativeFilterVariant=Disabled  NVariant=Disabled  NCopyVariant=Disabled_SignalSpec  FilterICVariant=Disabled  IntegratorICVariant=Disabled  ExternalResetVariant=Disabled  TRSumVariant=Passthrough  SumFdbkVariant=Disabled  SumVariant=Passthrough_P  TsampFilterVariant=InternalTs  TsampNgainVariant=Passthrough  TsampIntegralVariant=Disabled_SignalSpec
  Fix Faulty Baro : Saturate  UpperLimit=20  LowerLimit=-20
  Limit Output : Saturate  UpperLimit=0.9  LowerLimit=0.2
  Scale Vel : Gain  Gain=AltRateMax*2
  Sum1 : Sum  Inputs=|+-
  Sum3 : Sum  Inputs=|+-
  Thrust : Outport
  wires:
  Bias1/1 -> Limit Output/1  "VertVelOut5"
  Scale Vel/1 -> Sum3/1  "VertVelRef5"
  VertVel/1 -> Fix Faulty Baro/1
  Discrete PID Controller1/1 -> Bias1/1
  Sum3/1 -> Discrete PID Controller1/1
  AltRef/1 -> Sum1/1  "AltRef5"
  Altitude/1 -> Sum1/2
  Discrete PID Controller2/1 -> Scale Vel/1
  Sum1/1 -> Discrete PID Controller2/1
  Fix Faulty Baro/1 -> Sum3/2
  Limit Output/1 -> Thrust/1

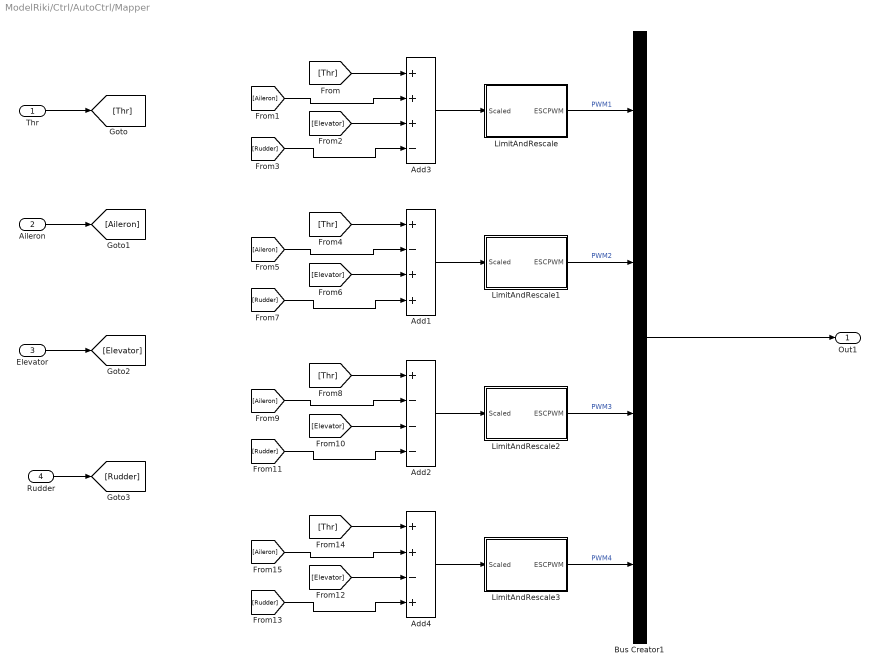
== system ModelRiki/Ctrl/AutoCtrl/Mapper ==
  Thr : Inport
  Aileron : Inport  Port=2
  Elevator : Inport  Port=3
  Rudder : Inport  Port=4
  Add1 : Sum  Inputs=+-++
  Add2 : Sum  Inputs=+---
  Add3 : Sum  Inputs=+++-
  Add4 : Sum  Inputs=++-+
  Bus Creator1 : BusCreator  Inputs=4
  LimitAndRescale : Subsystem
  LimitAndRescale1 : Subsystem
  LimitAndRescale2 : Subsystem
  LimitAndRescale3 : Subsystem
  Out1 : Outport
  wires:
  LimitAndRescale3/1(ESCPWM) -> Bus Creator1/4  "PWM4"
  Add4/1 -> LimitAndRescale3/1(Scaled)
  LimitAndRescale2/1(ESCPWM) -> Bus Creator1/3  "PWM3"
  Add2/1 -> LimitAndRescale2/1(Scaled)
  Bus Creator1/1 -> Out1/1
  LimitAndRescale/1(ESCPWM) -> Bus Creator1/1  "PWM1"
  Add3/1 -> LimitAndRescale/1(Scaled)
  LimitAndRescale1/1(ESCPWM) -> Bus Creator1/2  "PWM2"
  Thr/1 -> [Thr]
  Aileron/1 -> [Aileron]
  Elevator/1 -> [Elevator]
  Rudder/1 -> [Rudder]
  [Thr] -> Add3/1
  [Aileron] -> Add3/2
  [Elevator] -> Add3/3
  [Rudder] -> Add3/4
  Add1/1 -> LimitAndRescale1/1(Scaled)
  [Thr] -> Add1/1
  [Aileron] -> Add1/2
  [Elevator] -> Add1/3
  [Rudder] -> Add1/4
  [Thr] -> Add2/1
  [Aileron] -> Add2/2
  [Elevator] -> Add2/3
  [Rudder] -> Add2/4
  [Thr] -> Add4/1
  [Aileron] -> Add4/2
  [Elevator] -> Add4/3
  [Rudder] -> Add4/4
